simulink model "Admittance0x2DNEWWWW3"  (R2023b)
settings: Solver=FixedStepAuto  StartTime=0.0  StopTime=10.0  RelTol=1e-3
InitFcn:
  | J=1e-6
  | B = 1e-6
values from neighbouring files (symbols this model uses):
  K = 1.10e-4    (= 0.00011)    [Admittance_code.m]    (also in motor_model_state_space.m = 100)
  Ke = 0.011    [Admittance_code.m]    (also in motor_model_state_space.m)
  Kt = 0.011    [Admittance_code.m]    (also in motor_model_state_space.m)
  L = 0.58E-3    (= 0.00058)    [Admittance_code.m]    (also in motor_model_state_space.m)
  M_inv = 1/J    (= 617283.950617)    [Admittance_code.m]    (also in motor_model_state_space.m = 1000000)
  R = 1.17    [Admittance_code.m]    (also in motor_model_state_space.m)
libraries: slpidlib x1
settings Model: Creator=sayeholoumi  LastModifiedBy=sayeholoumi
settings OptimizationCC: DefaultParameterBehavior=Inlined  UseDivisionForNetSlopeComputation=on  GainParamInheritBuiltInType=on  UseFloatMulNetSlope=on  InlineInvariantSignals=on  PassReuseOutputArgsAs=Individual arguments  ZeroExternalMemoryAtStartup=off  ZeroInternalMemoryAtStartup=off  NoFixptDivByZeroProtection=on  EfficientFloat2IntCast=on  LifeSpan=1  OptimizeBlockOrder=speed  DifferentSizesBufferReuse=on  EfficientTunableParamExpr=on
settings DebuggingCC: ParameterTunabilityLossMsg=error
settings HardwareCC: ProdLongLongMode=on
settings SFSimCC: MATLABDynamicMemAlloc=off
settings RTWCC: Description=Embedded Coder  SystemTargetFile=ert.tlc  PackageGeneratedCodeAndArtifacts=on  TemplateMakefile=ert_default_tmf  TargetLang=C++
settings CodeAppCC: ForceParamTrailComments=on  IgnoreCustomStorageClasses=off  OperatorAnnotations=on  SimulinkDataObjDesc=on  SFDataObjDesc=on  CustomSymbolStrGlobalVar=rt$N$M  CustomSymbolStrType=$N$M  CustomSymbolStrFcn=$N$M$F  CustomSymbolStrMacro=$N$M  InsertBlockDesc=on
settings ERTTargetCC: TargetLangStandard=C++11 (ISO)  GenerateSampleERTMain=on  IncludeMdlTerminateFcn=off  CombineSignalStateStructs=on  SupportAbsoluteTime=off  CodeInterfacePackaging=C++ class  SupportComplex=off  SupportContinuousTime=on  InlinedParameterPlacement=NonHierarchical  RootIOFormat=Structure reference  ERTCustomFileTemplate=example_file_process.tlc  ERTFilePackagingFormat=CompactWithDataFile

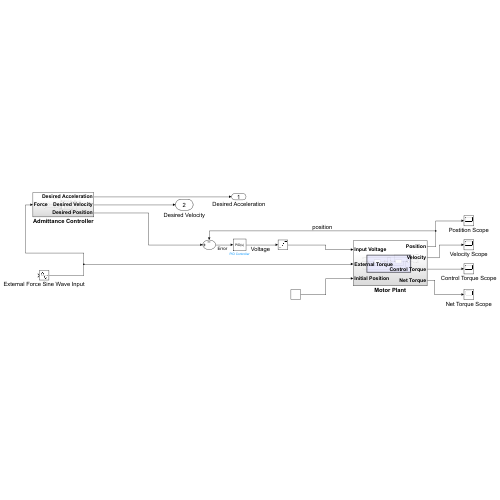
[thumbnail: Simulink's stored preview of the top-level diagram]
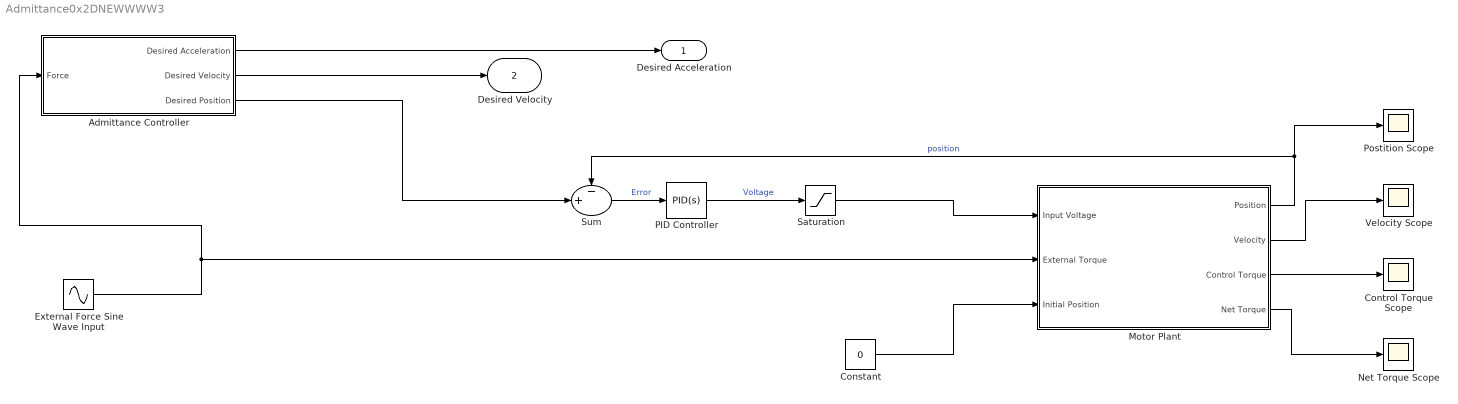
== system Admittance0x2DNEWWWW3 ==
  Admittance Controller : Subsystem
  Constant : Constant  Value=0
  Control Torque Scope : Scope
  External Force Sine Wave Input : Sin  TimeSource=Use external signal  SampleTime=0
  Motor Plant : Subsystem
  Net Torque Scope : Scope
  PID Controller : slpidlib/PID Controller  Controller=PID  Form=Parallel  TimeDomain=Continuous-time  UseExternalTs=off  SampleTime=-1  IntegratorMethod=Forward Euler  FilterMethod=Forward Euler  ControllerParametersSource=internal  P=1  I=1  UseKiTs=off  D=0  N=100  UseFilter=on  TunerSelectOption=Transfer Function Based (PID Tuner App)  InitialConditionSource=internal  InitialConditionForIntegrator=0  InitialConditionForFilter=0  DifferentiatorICPrevScaledInput=0  ExternalReset=none  TrackingMode=off  Kt=1  LimitOutput=off  SatLimitsSource=internal  UpperSaturationLimit=inf  LowerSaturationLimit=-inf  LinearizeAsGain=on  AntiWindupMode=none  Kb=1  LimitIntegrator=off  UpperIntegratorSaturationLimit=inf  LowerIntegratorSaturationLimit=-inf  POutMin=[]  POutMax=[]  IOutMin=[]  IOutMax=[]  DOutMin=[]  DOutMax=[]  NOutMin=[]  NOutMax=[]  SumOutMin=[]  SumOutMax=[]  SaturationOutMin=[]  SaturationOutMax=[]  PParamMin=[]  PParamMax=[]  IParamMin=[]  IParamMax=[]  DParamMin=[]  DParamMax=[]  NParamMin=[]  NParamMax=[]  KbParamMin=[]  KbParamMax=[]  KtParamMin=[]  KtParamMax=[]  KbOutMin=[]  KbOutMax=[]  KtOutMin=[]  KtOutMax=[]  IntegratorOutMin=[]  IntegratorOutMax=[]  FilterOutMin=[]  FilterOutMax=[]  SumI1OutMin=[]  SumI1OutMax=[]  SumI2OutMin=[]  SumI2OutMax=[]  SumI3OutMin=[]  SumI3OutMax=[]  SumI4OutMin=[]  SumI4OutMax=[]  SumDOutMin=[]  SumDOutMax=[]  DifferentiatorOutMin=[]  DifferentiatorOutMax=[]  FilterDiffOutCoefMin=[]  FilterDiffOutCoefMax=[]  ReciprocalOutMin=[]  ReciprocalOutMax=[]  SumDenOutMin=[]  SumDenOutMax=[]  SumNumOutMin=[]  SumNumOutMax=[]  DivideOutMin=[]  DivideOutMax=[]  UdiffTsProdOutMin=[]  UdiffTsProdOutMax=[]  NTsProdOutMin=[]  NTsProdOutMax=[]  UintegralTsProdOutMin=[]  UintegralTsProdOutMax=[]  UngainTsProdOutMin=[]  UngainTsProdOutMax=[]  ClampingZeroOutDataTypeStr=Inherit: Inherit via back propagation  ClampingZeroOutMin=[]  ClampingZeroOutMax=[]  FilterDenConstantOutDataTypeStr=Inherit: Inherit via back propagation  FilterDenConstantOutMin=[]  FilterDenConstantOutMax=[]  PCopyOutDataTypeStr=Inherit: Inherit via back propagation  PCopyOutMin=[]  PCopyOutMax=[]  NCopyOutDataTypeStr=Inherit: Inherit via back propagation  NCopyOutMin=[]  NCopyOutMax=[]  IntegratorContinuousStateAttributes=''  IntegratorStateMustResolveToSignalObject=off  IntegratorRTWStateStorageClass=Auto  FilterContinuousStateAttributes=''  FilterStateMustResolveToSignalObject=off  FilterRTWStateStorageClass=Auto  ParallelPVariant=InternalParameters  IdealPVariant=Disabled  IVariant=InternalParameters  DVariant=InternalParameters  IntegratorVariant=Continuous  SatVariant=Disabled  AWVariant=Passthrough  PCopyVariant=Disabled  TRVariant=Disabled  FdbkBlocksVariant=Forward  IdealPFdbkVariant=Disabled  SatFdbkVariant=Disabled  DerivativeFilterVariant=ContFilter  NVariant=InternalParameters  NCopyVariant=Disabled  FilterICVariant=InternalICsFilter  IntegratorICVariant=InternalICs  ExternalResetVariant=Disabled  TRSumVariant=Passthrough  SumFdbkVariant=Disabled  SumVariant=Sum_PID  TsampFilterVariant=InternalTs  TsampNgainVariant=Passthrough  TsampIntegralVariant=Disabled_SignalSpec  ExternalSaturationOutDataTypeStr=Inherit: Same as second input
  Postition Scope : Scope
  Saturation : Saturate  UpperLimit=12  LowerLimit=-12
  Sum : Sum  Inputs=-+|
  Velocity Scope : Scope
  Desired Acceleration : Outport
  Desired Velocity : Outport  Port=2
  wires:
  Admittance Controller/1(Desired Acceleration) -> Desired Acceleration/1
  Admittance Controller/3(Desired Position) -> Sum/2
  Admittance Controller/2(Desired Velocity) -> Desired Velocity/1
  Constant/1 -> Motor Plant/3(Initial Position)
  External Force Sine Wave Input/1 -> Admittance Controller/1(Force), Motor Plant/2(External Torque)
  Motor Plant/1(Position) -> Postition Scope/1, Sum/1  "position"
  PID Controller/1 -> Saturation/1  "Voltage"
  Motor Plant/4(Net Torque) -> Net Torque Scope/1
  Motor Plant/3(Control Torque) -> Control Torque Scope/1
  Saturation/1 -> Motor Plant/1(Input Voltage)
  Motor Plant/2(Velocity) -> Velocity Scope/1
  Sum/1 -> PID Controller/1  "Error"

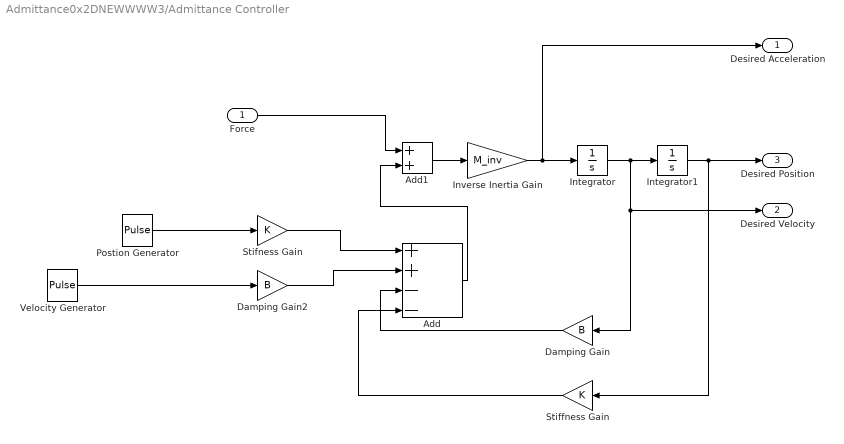
== system Admittance0x2DNEWWWW3/Admittance Controller ==
  Force : Inport
  Add : Sum  Inputs=++--
  Add1 : Sum
  Damping Gain : Gain  Gain=B
  Damping Gain2 : Gain  Gain=B
  Integrator : Integrator
  Integrator1 : Integrator
  Inverse Inertia Gain : Gain  Gain=M_inv
  Postion Generator : DiscretePulseGenerator  PulseType=Time based  Period=10  PulseWidth=5
  "Stiffness Gain " : Gain  Gain=K
  Stifness Gain : Gain  Gain=K
  Velocity Generator : DiscretePulseGenerator  PulseType=Time based  Period=10  PulseWidth=5
  Desired Acceleration : Outport
  Desired Velocity : Outport  Port=2
  Desired Position : Outport  Port=3
  wires:
  Postion Generator/1 -> Stifness Gain/1
  Damping Gain2/1 -> Add/2
  Add/1 -> Add1/2
  Add1/1 -> Inverse Inertia Gain/1
  Damping Gain/1 -> Add/3
  Inverse Inertia Gain/1 -> Desired Acceleration/1, Integrator/1
  "Stiffness Gain "/1 -> Add/4
  Integrator1/1 -> Desired Position/1, "Stiffness Gain "/1
  Stifness Gain/1 -> Add/1
  Force/1 -> Add1/1
  Integrator/1 -> Desired Velocity/1, Damping Gain/1, Integrator1/1
  Velocity Generator/1 -> Damping Gain2/1

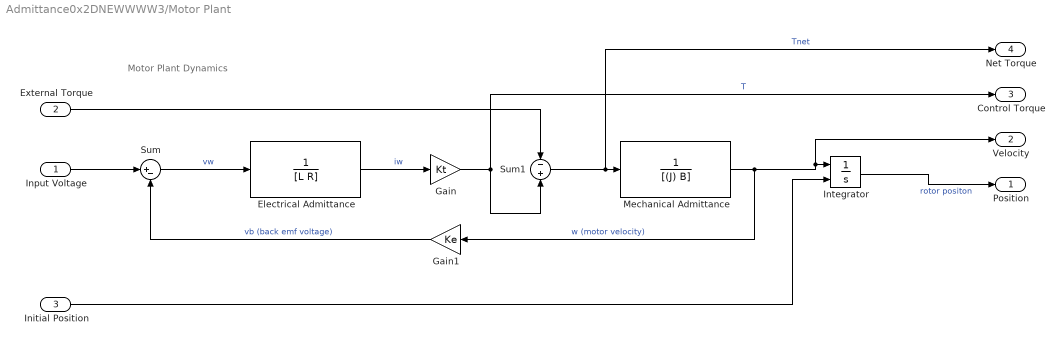
== system Admittance0x2DNEWWWW3/Motor Plant ==
  note: Motor Plant Dynamics
  Input Voltage : Inport
  External Torque : Inport  Port=2
  Initial Position : Inport  Port=3
  Electrical Admittance : TransferFcn  Denominator=[L R]
  Gain : Gain  Gain=Kt
  Gain1 : Gain  Gain=Ke
  Integrator : Integrator  InitialConditionSource=external
  Mechanical Admittance : TransferFcn  Denominator=[(J) B]
  Sum : Sum  Inputs=|+-
  Sum1 : Sum  Inputs=-+
  Position : Outport
  Velocity : Outport  Port=2
  Control Torque : Outport  Port=3
  Net Torque : Outport  Port=4
  wires:
  Input Voltage/1 -> Sum/1
  Mechanical Admittance/1 -> Velocity/1, Integrator/1, Gain1/1  "w (motor velocity)"
  Gain1/1 -> Sum/2  "vb (back emf voltage)"
  Integrator/1 -> Position/1  "rotor positon"
  Gain/1 -> Control Torque/1, Sum1/2  "T"
  Electrical Admittance/1 -> Gain/1  "iw"
  Sum/1 -> Electrical Admittance/1  "vw"
  Sum1/1 -> Net Torque/1, Mechanical Admittance/1  "Tnet"
  External Torque/1 -> Sum1/1
  Initial Position/1 -> Integrator/2
